simulink model "pid_discreto"  (R2021a)
settings: Solver=FixedStepAuto  StartTime=0.0  StopTime=10  FixedStep=T  RelTol=1e-3
values from neighbouring files (symbols this model uses):
  b = 1    [funcion_transferencia.m]
undefined symbols (not defined in the file or in its folder): a, DiscIntNeverNeededParam, Kp
settings Model: Creator=Bremdows  LastModifiedBy=Bremdows

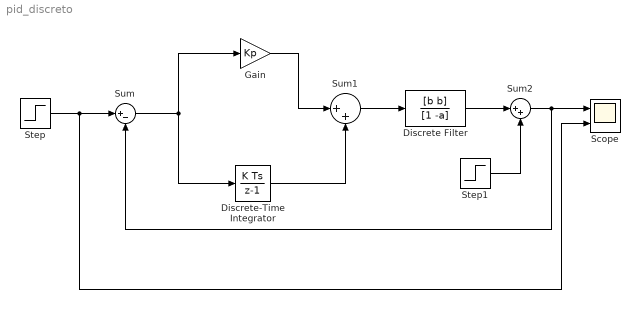
== system pid_discreto ==
  Discrete Filter : DiscreteFilter  Numerator=[b b]  Denominator=[1 -a]
  Discrete-Time Integrator : DiscreteIntegrator  gainval=5  SampleTime=-1  ICPrevOutput=DiscIntNeverNeededParam  ICPrevScaledInput=DiscIntNeverNeededParam
  Gain : Gain  Gain=Kp
  Scope : Scope  NumInputPorts=2
  Step : Step  Time=0
  Step1 : Step  Time=5  After=0.1
  Sum : Sum  Inputs=|+-
  Sum1 : Sum  Inputs=|++
  Sum2 : Sum  Inputs=|++
  wires:
  Discrete-Time Integrator/1 -> Sum1/2
  Gain/1 -> Sum1/1
  Sum1/1 -> Discrete Filter/1
  Step/1 -> Scope/2, Sum/1
  Sum/1 -> Discrete-Time Integrator/1, Gain/1
  Step1/1 -> Sum2/2
  Discrete Filter/1 -> Sum2/1
  Sum2/1 -> Sum/2, Scope/1
